simulink model "CLLC_WR"  (R2024a)
settings: Solver=ode4  StartTime=0.0  StopTime=0.2  FixedStep=1e-8  RelTol=1e-3
libraries: spsSeriesRLCBranchLib x9, spsVoltageMeasurementLib x7, spsMosfetLib x4, spsCurrentMeasurementLib x1, spsDCVoltageSourceLib x1, spsLinearTransformerLib x1, simulink x1, sps_lib x1
settings Model: Creator=Vishwajeet  LastModifiedBy=Vishwajeet

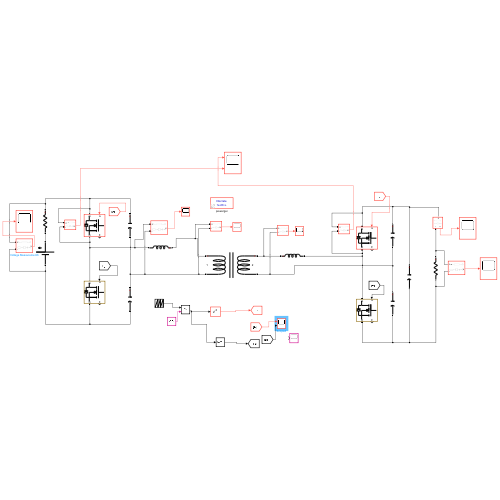
[thumbnail: Simulink's stored preview of the top-level diagram]
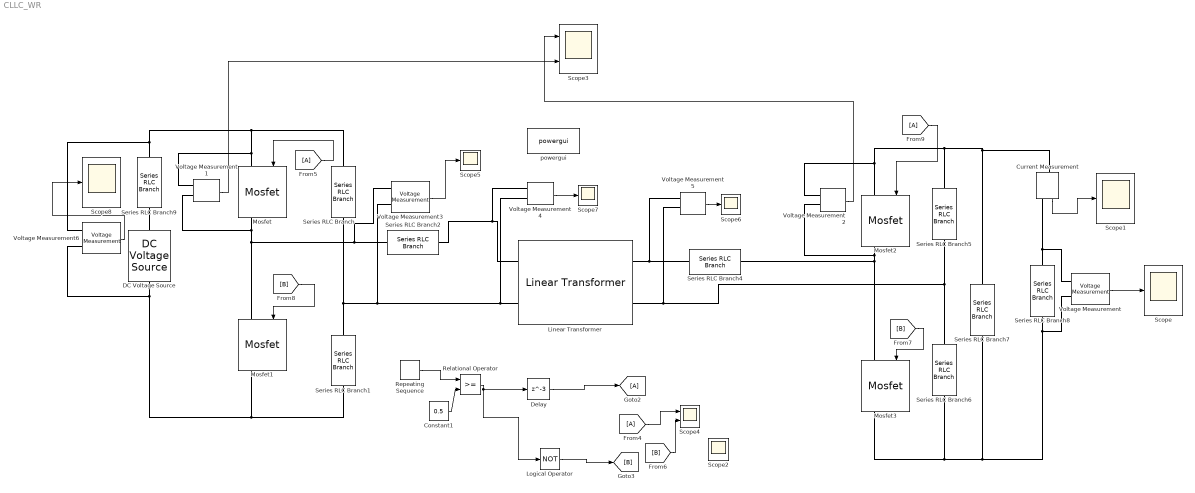
== system CLLC_WR ==
  Constant1 : Constant  Value=0.5
  Current Measurement : spsCurrentMeasurementLib/Current Measurement  PhasorSimulation=off  OutputType=Complex  PSBequivalent=0
  DC Voltage Source : spsDCVoltageSourceLib/DC Voltage Source  Amplitude=100  Measurements=Voltage
  Delay : Delay  DelayLength=3  InitialCondition=0
  From4 : From
  From5 : From
  From9 : From
  Goto2 : Goto
  Linear Transformer : spsLinearTransformerLib/Linear Transformer  UNITS=SI  NominalPower=[1.2e3 50]  winding1=[1 0 0]  winding2=[4 0 0]  ThreeWindings=off  winding3=[3.15e+05 1.9845e+05 50.535]  RmLm=[5e6 2.8e-6]  Measurements=None  DataType=on
  Logical Operator : Logic  Operator=NOT  AllPortsSameDT=off  OutDataTypeStr=boolean
  Mosfet{,1..3} (4 alike) : spsMosfetLib/Mosfet  Ron=0.1  Lon=0  Rd=0.01  Vfd=0  IC=0  Rs=1e5  Cs=inf  Measurements=on
  Relational Operator : RelationalOperator  OutDataTypeStr=boolean  RndMeth=Simplest  InputSameDT=off
  Repeating Sequence : simulink/Sources/Repeating Sequence  rep_seq_t=[0 40e-6]  rep_seq_y=[0 1]
  Scope{,1..2,5..8} (7 alike) : Scope
  Scope3 : Scope  NumInputPorts=2
  Scope4 : Scope  NumInputPorts=2
  Series RLC Branch{,1,5..6} (4 alike) : spsSeriesRLCBranchLib/Series RLC Branch  LConnTagsString=__new0  RConnTagsString=__new0  BranchType=C  Resistance=1  Inductance=1e-3  SetiL0=off  InitialCurrent=0  Capacitance=3.5e-6  Setx0=off  InitialVoltage=0  Measurements=None
  Series RLC Branch2 : spsSeriesRLCBranchLib/Series RLC Branch  LConnTagsString=__new0  RConnTagsString=__new0  BranchType=L  Resistance=1  Inductance=0.7e-6  SetiL0=off  InitialCurrent=0  Capacitance=1e-6  Setx0=off  InitialVoltage=0  Measurements=None
  Series RLC Branch4 : spsSeriesRLCBranchLib/Series RLC Branch  LConnTagsString=__new0  RConnTagsString=__new0  BranchType=L  Resistance=1  Inductance=0.7e-6  SetiL0=off  InitialCurrent=0  Capacitance=1e-6  Setx0=off  InitialVoltage=0  Measurements=None
  Series RLC Branch7 : spsSeriesRLCBranchLib/Series RLC Branch  LConnTagsString=__new0  RConnTagsString=__new0  BranchType=C  Resistance=1  Inductance=1e-3  SetiL0=off  InitialCurrent=0  Capacitance=1000e-6  Setx0=off  InitialVoltage=0  Measurements=None
  Series RLC Branch8 : spsSeriesRLCBranchLib/Series RLC Branch  LConnTagsString=__new0  RConnTagsString=__new0  BranchType=R  Resistance=160  Inductance=1e-3  SetiL0=off  InitialCurrent=0  Capacitance=1e-6  Setx0=off  InitialVoltage=0  Measurements=None
  Series RLC Branch9 : spsSeriesRLCBranchLib/Series RLC Branch  LConnTagsString=__new0  RConnTagsString=__new0  BranchType=R  Resistance=0.001  Inductance=1e-3  SetiL0=off  InitialCurrent=0  Capacitance=25.5-9  Setx0=off  InitialVoltage=0  Measurements=None
  Voltage Measurement{,1..6} (7 alike) : spsVoltageMeasurementLib/Voltage Measurement  PhasorSimulation=off  OutputType=Complex  PSBequivalent=0
  powergui : sps_lib/powergui  Priority=1  SimulationMode=Discrete  SampleTime=1e-8  frequency=60  Iterations=50  frequencyindice=0  Pbase=100e6  ErrMax=1e-4  UnitsV=kV  UnitsW=MW  buscounter=0  FunctionMessages=off  echomessages=off  EnableUseOfTLC=off  CurrentSourceSwitches=off  DisableSnubberDevices=off  DisableRonSwitches=off  DisableVfSwitches=off  DisplayEquations=off  AutomaticDiscreteSolvers=off  SolverType=Tustin/Backward Euler (TBE)  Interpol=off  ExternalGateDelay=off  methode=off  Ts=100  x0status=blocks  SPID=on  SwTol=0  HookPort=off  NonlinearTolerance=1e-4  nMaxIteration=100  ContinueOnMaxIteration=off  RestoreLinks=warning  ResistiveCurrentMeasurement=off  Frange=[0:2:500]  Ylog=off  Xlog=on  ShowGrid=off  save=off  variable=ZData  structure=0  ZoomFFT=off  StartTime=0.0  cycles=1  DisplayStyle=1  fundamental=60  FreqAxis=off  MaxFrequency=1000  frequencyindicesteady=1  RmsSteady=1  display=off
  wires:
  Current Measurement/1 -> Scope1/1
  Voltage Measurement/1 -> Scope/1
  Voltage Measurement2/1 -> Scope3/1
  Constant1/1 -> Relational Operator/2
  Repeating Sequence/1 -> Relational Operator/1
  From5/1 -> Mosfet/1
  [B] -> Mosfet3/1
  [B] -> Mosfet1/1
  From9/1 -> Mosfet2/1
  Voltage Measurement1/1 -> Scope3/2
  Voltage Measurement3/1 -> Scope5/1
  Logical Operator/1 -> [B]
  Voltage Measurement4/1 -> Scope7/1
  Delay/1 -> Goto2/1
  Relational Operator/1 -> Logical Operator/1, Delay/1
  Voltage Measurement5/1 -> Scope6/1
  From4/1 -> Scope4/1
  Voltage Measurement6/1 -> Scope8/1
  [B] -> Scope4/2
  connections:
  Mosfet1/LConn1 -- Voltage Measurement3/LConn1 -- Series RLC Branch2/RConn1 -- Voltage Measurement1/LConn2 -- Mosfet/RConn1
  Mosfet1/RConn1 -- Series RLC Branch1/RConn1 -- Voltage Measurement6/LConn2 -- DC Voltage Source/LConn1
  Mosfet/LConn1 -- Series RLC Branch/LConn1 -- Voltage Measurement6/LConn1 -- Series RLC Branch9/LConn1 -- Voltage Measurement1/LConn1
  Series RLC Branch1/LConn1 -- Voltage Measurement4/LConn2 -- Linear Transformer/LConn2 -- Voltage Measurement3/LConn2 -- Series RLC Branch/RConn1
  Series RLC Branch2/LConn1 -- Voltage Measurement4/LConn1 -- Linear Transformer/LConn1
  Series RLC Branch4/LConn1 -- Voltage Measurement5/LConn1 -- Linear Transformer/RConn1
  Mosfet3/LConn1 -- Series RLC Branch4/RConn1 -- Voltage Measurement2/LConn2 -- Mosfet2/RConn1
  Series RLC Branch8/LConn1 -- Current Measurement/RConn1 -- Voltage Measurement/LConn1
  Series RLC Branch8/RConn1 -- Mosfet3/RConn1 -- Series RLC Branch6/RConn1 -- Series RLC Branch7/RConn1 -- Voltage Measurement/LConn2
  Series RLC Branch7/LConn1 -- Voltage Measurement2/LConn1 -- Mosfet2/LConn1 -- Series RLC Branch5/LConn1 -- Current Measurement/LConn1
  Series RLC Branch6/LConn1 -- Voltage Measurement5/LConn2 -- Linear Transformer/RConn2 -- Series RLC Branch5/RConn1
  Series RLC Branch9/RConn1 -- DC Voltage Source/RConn1
